simulink model "ysw3_25"  (R2014a)
settings: Solver=ode45  StartTime=0.0  StopTime=10.0  RelTol=1e-3
settings Model: Creator=Administrator  LastModifiedBy=Administrator

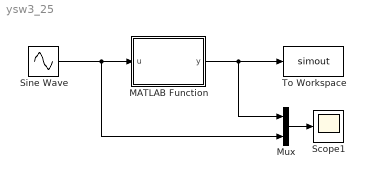
== system ysw3_25 ==
  MATLAB Function : MATLAB Function  TreatAsAtomicUnit=on
  Mux : Mux  Inputs=2
  Scope1 : Scope
      settings: TimeRange=10
  Sine Wave : Sin  SampleTime=0.1
  To Workspace : ToWorkspace  VariableName=simout  SaveFormat=Timeseries  SampleTime=-1
  wires:
  Mux/1 -> Scope1/1
  Sine Wave/1 -> MATLAB Function/1(u), Mux/2
  MATLAB Function/1(y) -> Mux/1, To Workspace/1

== matlab function ysw3_25/MATLAB Function ==
  data: u input; y output
function y = fcn(u)
%#codegen
y = sin(u)*cos(u).^.2+exp(sin(u));
